simulink model "sgMdl_IO643_IO644_CANopenLoopback"  (R2024b)
settings: Solver=FixedStepAuto  StartTime=0.0  StopTime=inf  RelTol=1e-3  EnableMultiTasking=on
undefined symbols (not defined in the file): Ts, ts
libraries: speedgoatlib_IO644 x16, slrealtimeutilitieslib x6, speedgoatlib_IO643 x6, simulink x6, speedgoatlib_shared x1
Description:
  | IO643 & IO644 - CANopen Loopback
settings Model: ModifiedByFormat=Speedgoat  Creator=Speedgoat  LastModifiedBy=Speedgoat
settings SolverCC: ConcurrentTasks=on  AlgebraicLoopSolver=TrustRegion  PositivePriorityOrder=on  AutoInsertRateTranBlk=on  InsertRTBMode=Never (minimum delay)
settings DataIOCC: SaveFormat=Array  SaveState=on  SignalLoggingName=logsOut
settings OptimizationCC: BlockReduction=off  BooleanDataType=off  OptimizeBlockIOStorage=off  BufferReuse=off  GlobalBufferReuse=off  ExpressionFolding=off  LocalBlockOutputs=off  InitFltsAndDblsToZero=on  OptimizeDataStoreBuffers=off  BusAssignmentInplaceUpdate=off
settings DebuggingCC: SaveWithParameterizedLinksMsg=none  UnderspecifiedInitializationDetection=Classic  MergeDetectMultiDrivingBlocksExec=none  CheckExecutionContextPreStartOutputMsg=on  SignalResolutionControl=TryResolveAllWithWarning  TasksWithSamePriorityMsg=none  UnconnectedInputMsg=warning  UnconnectedOutputMsg=warning  UnconnectedLineMsg=warning  SFUnexpectedBacktrackingDiag=warning  SFNoUnconditionalDefaultTransitionDiag=warning  SFExecutionAtInitializationDiag=none  ArithmeticOperatorsInVariantConditions=warning
settings HardwareCC: ProdBitPerLong=64  ProdLongLongMode=on  ProdHWDeviceType=Intel->x86-64 (Linux 64)
settings ModelReferenceCC: EnableRefExpFcnMdlSchedulingChecks=on  PropagateSignalLabelsOutOfModel=off
settings SFSimCC: SimUseLocalCustomCode=off  SimTargetLang=C++
settings RTWCC: Description=Speedgoat Real-Time Target Machine  SystemTargetFile=speedgoat.tlc  TemplateMakefile=slrealtime_default_tmf  RTWUseLocalCustomCode=off  Toolchain=Simulink Real-Time Toolchain  BuildConfiguration=Faster Runs  TargetLang=C++  GPUComputeCapability=3.5  DLArmComputeVersion=19.05
settings CodeAppCC: StateflowObjectComments=on
settings SimulinkRealTimeTargetCC: SubcomponentCodeInterfacePackaging=Reusable function  InstructionSetFMA=off  LogToMDFFile=off  SLRTFileLogMaxRuns=10
settings ConfigComp: CovMetricSettings=dw  CovSaveCumulativeToWorkspaceVar=on  CovSaveSingleToWorkspaceVar=on  CovExternalEMLEnable=off  CovSFcnEnable=off  CovBoundaryAbsTol=1.0e-5

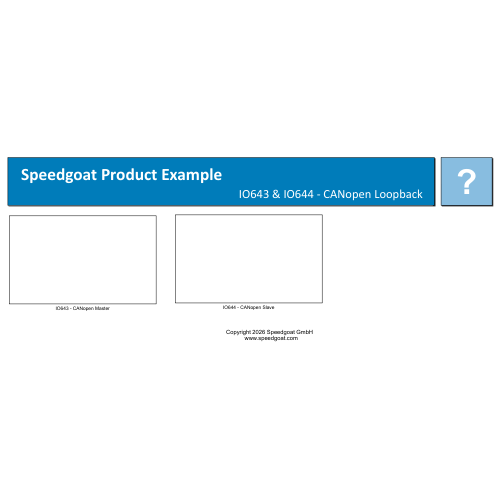
[thumbnail: Simulink's stored preview of the top-level diagram]
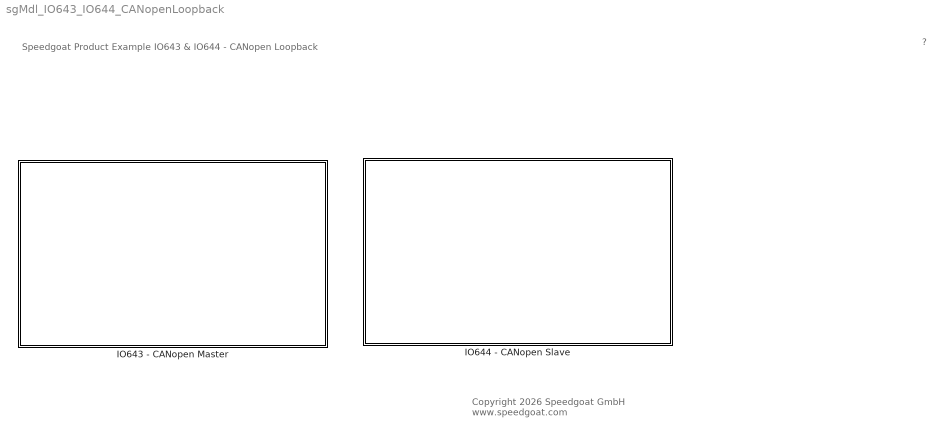
== system sgMdl_IO643_IO644_CANopenLoopback ==
  note: Speedgoat Product Example
      | IO643 & IO644 - CANopen Loopback
  note: ?
  note: Copyright 2026 Speedgoat GmbH
      |  www.speedgoat.com
  IO643 - CANopen Master : Subsystem
  IO644 - CANopen Slave : Subsystem

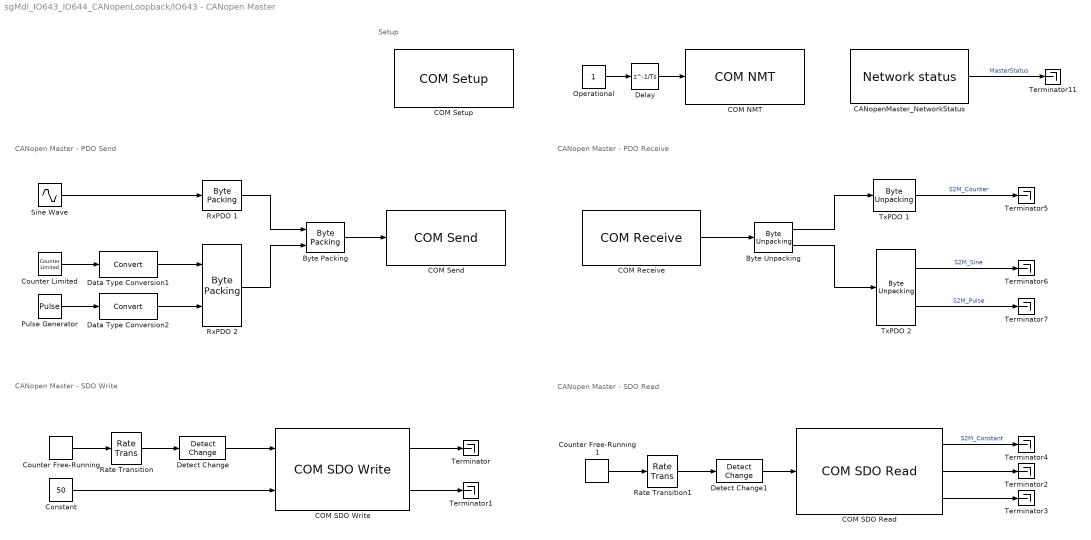
== system sgMdl_IO643_IO644_CANopenLoopback/IO643 - CANopen Master ==
  note: CANopen Master - SDO Write
  note: CANopen Master - PDO Send
  note: CANopen Master - PDO Receive
  note: Setup
  note: CANopen Master - SDO Read
  Byte Packing : slrealtimeutilitieslib/Byte Packing  MaskPackedDataType=uint8  MaskUnpackedDataTypes={'uint8','uint8'}  MaskAlignment=1
  Byte Unpacking : slrealtimeutilitieslib/Byte Unpacking  MaskUnpackedDataTypes={'uint8','uint8'}  MaskUnpackedDataSizes={[4],[5]}  MaskAlignment=1
  CANopenMaster_NetworkStatus : speedgoatlib_shared/IO75X/Network status  id=1  get_status=on  set_status=off  timeout=0.01  ts=Ts
  COM NMT : speedgoatlib_IO643/COM NMT  id=1  CanNodeId=2  SampleTime=Ts
      settings: SourceProductName=IO643 CANopen Master
  COM Receive : speedgoatlib_IO643/COM Receive  id=1  parDataLen=9  parSampleTime=Ts
      settings: SourceProductName=IO643 CANopen Master
  COM SDO Read : speedgoatlib_IO643/COM SDO Read  id=1  CanNodeId=2  SdoIndex=hex2dec('4000')  SdoSubIndex=0  InitValue=int16(0)  SampleTime=Ts
      settings: SourceProductName=IO643 CANopen Master
  COM SDO Write : speedgoatlib_IO643/COM SDO Write  id=1  CanNodeId=2  SdoIndex=hex2dec('6000')  SdoSubIndex=0  SampleTime=Ts
      settings: SourceProductName=IO643 CANopen Master
  COM Send : speedgoatlib_IO643/COM Send  id=1  parDataLen=14  parSampleTime=Ts
      settings: SourceProductName=IO643 CANopen Master
  COM Setup : speedgoatlib_IO643/COM Setup  id=1  BusSlot=-1  HostFile=which('IO643_IO644_Loopback_m.nxd')
      settings: SourceProductName=IO643 CANopen Master
  Constant : Constant  Value=50  OutDataTypeStr=int8  SampleTime=Ts
  Counter Free-Running : simulink/Sources/Counter Free-Running  NumBits=16  tsamp=1
  Counter Free-Running1 : simulink/Sources/Counter Free-Running  NumBits=16  tsamp=1
  Counter Limited : simulink/Sources/Counter Limited  uplimit=100  tsamp=Ts/Ts/10
  Data Type Conversion1 : DataTypeConversion  SaturateOnIntegerOverflow=off  RndMeth=Floor
  Data Type Conversion2 : DataTypeConversion  SaturateOnIntegerOverflow=off  RndMeth=Floor
  Delay : Delay  DelayLength=1/Ts
  Detect Change : simulink/Logic and Bit Operations/Detect Change  vinit=0  OutDataTypeStr=boolean
  Detect Change1 : simulink/Logic and Bit Operations/Detect Change  vinit=0  OutDataTypeStr=boolean
  Operational : Constant  OutDataTypeStr=Inherit: Inherit via back propagation
  Pulse Generator : DiscretePulseGenerator  Amplitude=100  Period=2*1/Ts  PulseWidth=1/Ts  SampleTime=Ts
  Rate Transition : RateTransition
  Rate Transition1 : RateTransition
  RxPDO 1 : slrealtimeutilitieslib/Byte Packing  MaskPackedDataType=uint8  MaskUnpackedDataTypes={'double'}  MaskAlignment=1
  RxPDO 2 : slrealtimeutilitieslib/Byte Packing  MaskPackedDataType=uint8  MaskUnpackedDataTypes={'uint16','int32'}  MaskAlignment=1
  Sine Wave : Sin  Amplitude=100  Frequency=2*pi  Phase=pi  SampleTime=Ts
  Terminator{,1..7,11} (9 alike) : Terminator
  TxPDO 1 : slrealtimeutilitieslib/Byte Unpacking  MaskUnpackedDataTypes={'uint32'}  MaskUnpackedDataSizes={[1]}  MaskAlignment=1
  TxPDO 2 : slrealtimeutilitieslib/Byte Unpacking  MaskUnpackedDataTypes={'single','uint8'}  MaskUnpackedDataSizes={[1],[1]}  MaskAlignment=1
  wires:
  Sine Wave/1 -> RxPDO 1/1
  Counter Limited/1 -> Data Type Conversion1/1
  Constant/1 -> COM SDO Write/2
  COM SDO Read/1 -> Terminator4/1  "S2M_Constant"
  TxPDO 1/1 -> Terminator5/1  "S2M_Counter"
  TxPDO 2/1 -> Terminator6/1  "S2M_Sine"
  TxPDO 2/2 -> Terminator7/1  "S2M_Pulse"
  Data Type Conversion1/1 -> RxPDO 2/1
  Data Type Conversion2/1 -> RxPDO 2/2
  Byte Packing/1 -> COM Send/1
  Pulse Generator/1 -> Data Type Conversion2/1
  CANopenMaster_NetworkStatus/1 -> Terminator11/1  "MasterStatus"
  RxPDO 2/1 -> Byte Packing/2
  RxPDO 1/1 -> Byte Packing/1
  Byte Unpacking/2 -> TxPDO 2/1
  COM Receive/1 -> Byte Unpacking/1
  Byte Unpacking/1 -> TxPDO 1/1
  Detect Change/1 -> COM SDO Write/1
  COM SDO Write/1 -> Terminator/1
  COM SDO Write/2 -> Terminator1/1
  COM SDO Read/2 -> Terminator2/1
  COM SDO Read/3 -> Terminator3/1
  Counter Free-Running/1 -> Rate Transition/1
  Rate Transition/1 -> Detect Change/1
  Rate Transition1/1 -> Detect Change1/1
  Counter Free-Running1/1 -> Rate Transition1/1
  Detect Change1/1 -> COM SDO Read/1
  Operational/1 -> Delay/1
  Delay/1 -> COM NMT/1

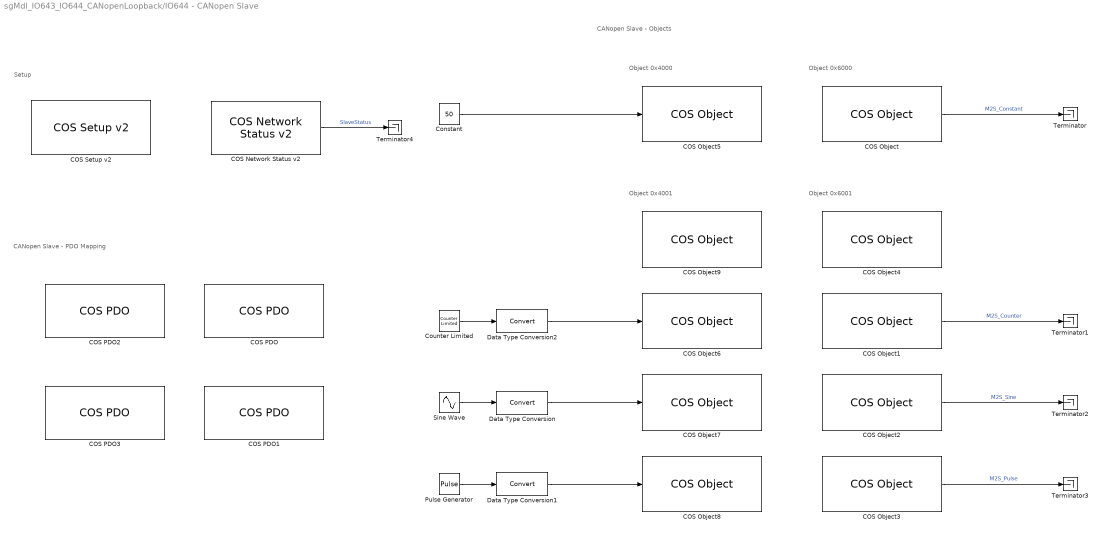
== system sgMdl_IO643_IO644_CANopenLoopback/IO644 - CANopen Slave ==
  note: CANopen Slave - PDO Mapping
  note: Object 0x6001
  note: CANopen Slave - Objects
  note: Setup
  note: Object 0x6000
  note: Object 0x4000
  note: Object 0x4001
  COS Network Status v2 : speedgoatlib_IO644/COS Network Status v2  id=2  StateControl=off  StateCommand=off  ExtDiag=off  Monitoring=off  SampleTime=Ts
      settings: SourceProductName=IO644 CANopen Slave
  COS Object : speedgoatlib_IO644/COS Object  id=2  ObjectName='M2S_Constant'  Index=0x6000  SubIndex=0  ObjectType=VAR  DataType=INTEGER8  AccessRights=rw  InitValue=int8(0)  ReadOp=on  WriteOp=off  ExtendedInterface=off  SampleTime=Ts
      settings: SourceProductName=IO644 CANopen Slave
      settings: AttributesFormatString=|
      | %<Index>
      | %<ObjectName>
  COS Object1 : speedgoatlib_IO644/COS Object  id=2  ObjectName='M2S_Counter'  Index=0x6001  SubIndex=1  ObjectType=VAR  DataType=USIGNED16  AccessRights=wo  InitValue=uint16(0)  ReadOp=on  WriteOp=off  ExtendedInterface=off  SampleTime=Ts
      settings: SourceProductName=IO644 CANopen Slave
      settings: AttributesFormatString=|
      | %<Index>:%<SubIndex>
      | %<ObjectName>
  COS Object2 : speedgoatlib_IO644/COS Object  id=2  ObjectName='M2S_Sine'  Index=0x6001  SubIndex=2  ObjectType=VAR  DataType=REAL64  AccessRights=wo  InitValue=double(0)  ReadOp=on  WriteOp=off  ExtendedInterface=off  SampleTime=Ts
      settings: SourceProductName=IO644 CANopen Slave
      settings: AttributesFormatString=|
      | %<Index>:%<SubIndex>
      | %<ObjectName>
  COS Object3 : speedgoatlib_IO644/COS Object  id=2  ObjectName='M2S_Pulse'  Index=0x6001  SubIndex=3  ObjectType=VAR  DataType=INTEGER32  AccessRights=wo  InitValue=int32(0)  ReadOp=on  WriteOp=off  ExtendedInterface=off  SampleTime=Ts
      settings: SourceProductName=IO644 CANopen Slave
      settings: AttributesFormatString=|
      | %<Index>:%<SubIndex>
      | %<ObjectName>
  COS Object4 : speedgoatlib_IO644/COS Object  id=2  ObjectName='Object_2'  Index=0x6001  SubIndex=0  ObjectType=RECORD  DataType=USIGNED16  AccessRights=wo  InitValue=uint16(0)  ReadOp=off  WriteOp=off  ExtendedInterface=off  SampleTime=Ts
      settings: SourceProductName=IO644 CANopen Slave
      settings: AttributesFormatString=|
      | %<Index>
      | %<ObjectName>
  COS Object5 : speedgoatlib_IO644/COS Object  id=2  ObjectName='S2M_Constant'  Index=0x4000  SubIndex=0  ObjectType=VAR  DataType=INTEGER16  AccessRights=rw  InitValue=int16(0)  ReadOp=off  WriteOp=on  ExtendedInterface=off  SampleTime=Ts
      settings: SourceProductName=IO644 CANopen Slave
      settings: AttributesFormatString=|
      | %<Index>
      | %<ObjectName>
  COS Object6 : speedgoatlib_IO644/COS Object  id=2  ObjectName='S2M_Counter'  Index=0x4001  SubIndex=1  ObjectType=VAR  DataType=USIGNED32  AccessRights=ro  InitValue=uint32(0)  ReadOp=off  WriteOp=on  ExtendedInterface=off  SampleTime=Ts
      settings: SourceProductName=IO644 CANopen Slave
      settings: AttributesFormatString=|
      | %<Index>:%<SubIndex>
      | %<ObjectName>
  COS Object7 : speedgoatlib_IO644/COS Object  id=2  ObjectName='S2M_Sine'  Index=0x4001  SubIndex=2  ObjectType=VAR  DataType=REAL32  AccessRights=ro  InitValue=single(0)  ReadOp=off  WriteOp=on  ExtendedInterface=off  SampleTime=Ts
      settings: SourceProductName=IO644 CANopen Slave
      settings: AttributesFormatString=|
      | %<Index>:%<SubIndex>
      | %<ObjectName>
  COS Object8 : speedgoatlib_IO644/COS Object  id=2  ObjectName='S2M_Pulse'  Index=0x4001  SubIndex=3  ObjectType=VAR  DataType=USIGNED8  AccessRights=ro  InitValue=uint8(5)  ReadOp=off  WriteOp=on  ExtendedInterface=off  SampleTime=Ts
      settings: SourceProductName=IO644 CANopen Slave
      settings: AttributesFormatString=|
      | %<Index>:%<SubIndex>
      | %<ObjectName>
  COS Object9 : speedgoatlib_IO644/COS Object  id=2  ObjectName='Object_1'  Index=0x4001  SubIndex=0  ObjectType=RECORD  DataType=USIGNED16  AccessRights=wo  InitValue=uint16(0)  ReadOp=off  WriteOp=off  ExtendedInterface=off  SampleTime=Ts
      settings: SourceProductName=IO644 CANopen Slave
      settings: AttributesFormatString=|
      | %<Index>
      | %<ObjectName>
  COS PDO : speedgoatlib_IO644/COS PDO  id=2  SampleTime=ts  PdoType=Rx  PdoId=1  CobId=0  Mapping=[0x6001,2]  TransType=synchronous cyclic  TransRate=1  InhibitTime=0  EventTimer=0  SyncStartValue=0
      settings: SourceProductName=IO644 CANopen Slave
      settings: AttributesFormatString=|
      | %<PdoType>PDO %<PdoId>
      | %<Mapping>
  COS PDO1 : speedgoatlib_IO644/COS PDO  id=2  SampleTime=ts  PdoType=Rx  PdoId=2  CobId=0  Mapping=[0x6001,1;0x6001,3]  TransType=event-driven manufacturer specific  TransRate=1  InhibitTime=0  EventTimer=0  SyncStartValue=0
      settings: SourceProductName=IO644 CANopen Slave
      settings: AttributesFormatString=|
      | %<PdoType>PDO %<PdoId>
      | %<Mapping>
  COS PDO2 : speedgoatlib_IO644/COS PDO  id=2  SampleTime=ts  PdoType=Tx  PdoId=1  CobId=0  Mapping=[0x4001,1]  TransType=event-driven manufacturer specific  TransRate=1  InhibitTime=0  EventTimer=50  SyncStartValue=0
      settings: SourceProductName=IO644 CANopen Slave
      settings: AttributesFormatString=|
      | %<PdoType>PDO %<PdoId>
      | %<Mapping>
  COS PDO3 : speedgoatlib_IO644/COS PDO  id=2  SampleTime=ts  PdoType=Tx  PdoId=2  CobId=0  Mapping=[0x4001,2;0x4001,3]  TransType=synchronous cyclic  TransRate=1  InhibitTime=0  EventTimer=1  SyncStartValue=0
      settings: SourceProductName=IO644 CANopen Slave
      settings: AttributesFormatString=|
      | %<PdoType>PDO %<PdoId>
      | %<Mapping>
  COS Setup v2 : speedgoatlib_IO644/COS Setup v2  id=2  PciBusSlot=-1  CanNodeID=2  BaudRate=Auto  DeviceType=0  VendorName='Speedgoat'  VendorId=0x00000267  ProductName='IO644'  ProductCode=1  RevNum=1  HbProducer=0  HbConsumer=[]  GuardTime=0  LifeTimeFactor=0
      settings: SourceProductName=IO644 CANopen Slave
  Constant : Constant  Value=50  OutDataTypeStr=Inherit: Inherit via back propagation  SampleTime=Ts
  Counter Limited : simulink/Sources/Counter Limited  uplimit=100  tsamp=0.1
  Data Type Conversion : DataTypeConversion  SaturateOnIntegerOverflow=off  RndMeth=Floor
  Data Type Conversion1 : DataTypeConversion  SaturateOnIntegerOverflow=off  RndMeth=Floor
  Data Type Conversion2 : DataTypeConversion  SaturateOnIntegerOverflow=off  RndMeth=Floor
  Pulse Generator : DiscretePulseGenerator  Amplitude=100  Period=2*1/Ts  PulseWidth=1/Ts  SampleTime=Ts
  Sine Wave : Sin  Amplitude=100  Frequency=2*pi  Phase=pi  SampleTime=Ts
  Terminator{,1..4} (5 alike) : Terminator
  wires:
  COS Object/1 -> Terminator/1  "M2S_Constant"
  COS Object1/1 -> Terminator1/1  "M2S_Counter"
  COS Object2/1 -> Terminator2/1  "M2S_Sine"
  COS Object3/1 -> Terminator3/1  "M2S_Pulse"
  Constant/1 -> COS Object5/1
  Counter Limited/1 -> Data Type Conversion2/1
  Sine Wave/1 -> Data Type Conversion/1
  Data Type Conversion/1 -> COS Object7/1
  Data Type Conversion1/1 -> COS Object8/1
  Data Type Conversion2/1 -> COS Object6/1
  Pulse Generator/1 -> Data Type Conversion1/1
  COS Network Status v2/1 -> Terminator4/1  "SlaveStatus"
